simulink model "ACCnovis"  (R2018b)
settings: Solver=ode45  StartTime=0.0  StopTime=80  RelTol=1e-3  EnableMultiTasking=on
values from neighbouring files (symbols this model uses):
  h = 0.9    [initialization.m]
  Kd = 1.2    [initialization.m]
  Kp = 1.5    [initialization.m]
  Lambda1 = 0.5    [initialization.m]
  Lambda2 = 0.7    [initialization.m]
  Lambda3 = 0.75    [initialization.m]
  Lambda4 = 0.7    [initialization.m]
  Lambda5 = 0.7    [initialization.m]
  tau0 = 0.1    [initialization.m]
  tau1 = 0.5    [initialization.m]
  tau2 = 0.7    [initialization.m]
  tau3 = 0.3    [initialization.m]
  tau4 = 0.7    [initialization.m]
  tau5 = 0.9    [initialization.m]
undefined symbols (not defined in the file or in its folder): sigbuilder_block
libraries: simulink x5
settings Model: Creator=apple  LastModifiedBy=ajink
settings DataIOCC: LimitDataPoints=on  SaveFormat=Array
settings OptimizationCC: LifeSpan=inf
settings DebuggingCC: SFUnexpectedBacktrackingDiag=warning  SFNoUnconditionalDefaultTransitionDiag=warning  SFExecutionAtInitializationDiag=none
settings HardwareCC: ProdBitPerPointer=32  ProdBitPerSizeT=32  ProdBitPerPtrDiffT=32  ProdLargestAtomicFloat=None  ProdIntDivRoundTo=Undefined  ProdEndianess=Unspecified  ProdWordSize=32  ProdHWDeviceType=32-bit Generic
settings ModelReferenceCC: PropagateSignalLabelsOutOfModel=off
settings SFSimCC: SimUseLocalCustomCode=off
settings RTWCC: RTWUseLocalCustomCode=off
settings CodeAppCC: StateflowObjectComments=on
settings GRTTargetCC: TargetLangStandard=C89/C90 (ANSI)  GeneratePreprocessorConditionals=Disable all
settings ConfigComp: CovMetricSettings=dw  CovHtmlReporting=on  CovSaveCumulativeToWorkspaceVar=on  CovSaveSingleToWorkspaceVar=on  CovExternalEMLEnable=off

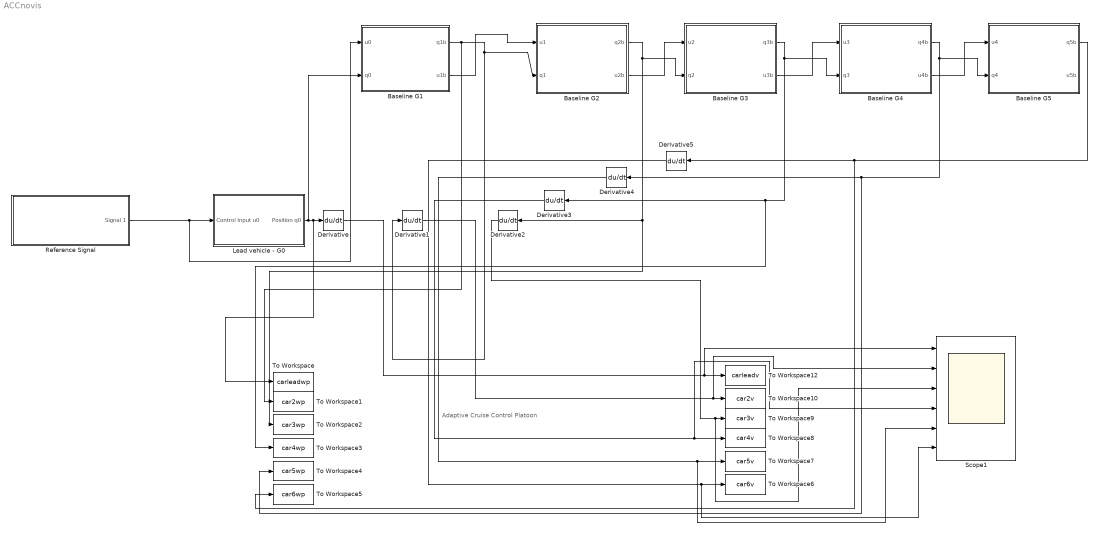
== system ACCnovis ==
  note: Adaptive Cruise Control Platoon
  Baseline G1 : Subsystem
  Baseline G2 : Subsystem
  Baseline G3 : Subsystem
  Baseline G4 : Subsystem
  Baseline G5 : Subsystem
  Derivative{,1..5} (6 alike) : Derivative
  Lead vehicle - G0 : Subsystem
  Reference Signal : Subsystem  Tag=STV Subsys  LoadFcn=sigbuilder_block('load');  StartFcn=sigbuilder_block('start');  StopFcn=sigbuilder_block('stop');  ClipboardFcn=sigbuilder_block('clipboard');  mask(Sigbuilder block){tuvar=[0:10]}
      mask help: Simulink:masks:SigbuilderBlock_MD
      mask init:
      | if ~strcmp(get_param(bdroot(gcbh),'SimulationStatus'),'stopped') tuvar = sigbuilder_block('maskInit'); end
      settings: CopyFcn=sigbuilder_block('copy');  DeleteFcn=sigbuilder_block('delete');  ModelCloseFcn=sigbuilder_block('modelClose');  PreSaveFcn=sigbuilder_block('preSave');  PauseFcn=sigbuilder_block('pause');  ContinueFcn=sigbuilder_block('continue');  NameChangeFcn=sigbuilder_block('namechange');  OpenFcn=sigbuilder_block('open',[6 30 948 639.75 ]);  CloseFcn=sigbuilder_block('close');
      mask Display: plot(0, 0, 100, 100,[2, 2, 32, 32, 2], [68, 8, 8, 68, 68],[32, 2], [38, 38], [32, 19, 2],[53, 60, 44], [32, 17, 17, 2],[16, 16, 31, 31]);txt = getActiveGroup(gcbh);text(2, 100, txt,'verticalAlignment', 'top');
  Scope1 : Scope  NumInputPorts=6
  To Workspace : ToWorkspace  VariableName=carleadwp  SampleTime=-1
      settings: Save2DSignal=2-D array (concatenate along first dimension)
  To Workspace1 : ToWorkspace  VariableName=car2wp  SampleTime=-1
      settings: Save2DSignal=2-D array (concatenate along first dimension)
  To Workspace10 : ToWorkspace  VariableName=car2v  SampleTime=-1
      settings: Save2DSignal=2-D array (concatenate along first dimension)
  To Workspace12 : ToWorkspace  VariableName=carleadv  SampleTime=-1
      settings: Save2DSignal=2-D array (concatenate along first dimension)
  To Workspace2 : ToWorkspace  VariableName=car3wp  SampleTime=-1
      settings: Save2DSignal=2-D array (concatenate along first dimension)
  To Workspace3 : ToWorkspace  VariableName=car4wp  SampleTime=-1
      settings: Save2DSignal=2-D array (concatenate along first dimension)
  To Workspace4 : ToWorkspace  VariableName=car5wp  SampleTime=-1
      settings: Save2DSignal=2-D array (concatenate along first dimension)
  To Workspace5 : ToWorkspace  VariableName=car6wp  SampleTime=-1
      settings: Save2DSignal=2-D array (concatenate along first dimension)
  To Workspace6 : ToWorkspace  VariableName=car6v  SampleTime=-1
      settings: Save2DSignal=2-D array (concatenate along first dimension)
  To Workspace7 : ToWorkspace  VariableName=car5v  SampleTime=-1
      settings: Save2DSignal=2-D array (concatenate along first dimension)
  To Workspace8 : ToWorkspace  VariableName=car4v  SampleTime=-1
      settings: Save2DSignal=2-D array (concatenate along first dimension)
  To Workspace9 : ToWorkspace  VariableName=car3v  SampleTime=-1
      settings: Save2DSignal=2-D array (concatenate along first dimension)
  wires:
  Reference Signal/1(Signal 1) -> Baseline G1/1(u0), Lead vehicle - G0/1(Control Input u0)
  Lead vehicle - G0/1(" Position q0") -> Baseline G1/2(q0), To Workspace/1, Derivative/1
  Baseline G1/1(q1b) -> To Workspace1/1, Baseline G2/2(q1), Derivative1/1
  Derivative/1 -> Scope1/1, To Workspace12/1
  Derivative1/1 -> Scope1/2, To Workspace10/1
  Baseline G1/2(u1b) -> Baseline G2/1(u1)
  Baseline G2/1(q2b) -> To Workspace2/1, Derivative2/1, Baseline G3/2(q2)
  Derivative2/1 -> Scope1/3, To Workspace9/1
  Baseline G2/2(u2b) -> Baseline G3/1(u2)
  Baseline G3/1(q3b) -> Baseline G4/2(q3), To Workspace3/1, Derivative3/1
  Derivative3/1 -> Scope1/4, To Workspace8/1
  Baseline G3/2(u3b) -> Baseline G4/1(u3)
  Baseline G4/1(q4b) -> Baseline G5/2(q4), To Workspace4/1, Derivative4/1
  Derivative4/1 -> Scope1/5, To Workspace7/1
  Baseline G4/2(u4b) -> Baseline G5/1(u4)
  Baseline G5/1(q5b) -> To Workspace5/1, Derivative5/1
  Derivative5/1 -> Scope1/6, To Workspace6/1

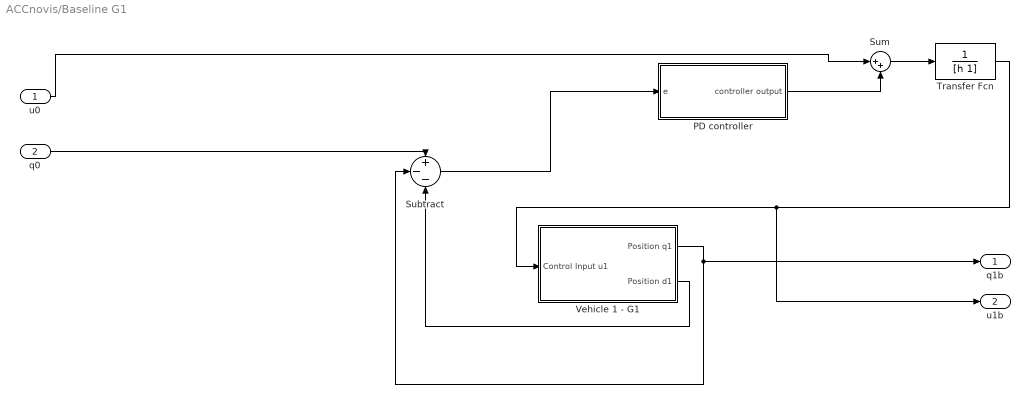
== system ACCnovis/Baseline G1 ==
  u0 : Inport
  q0 : Inport  Port=2
  PD controller : Subsystem
  Subtract : Sum  Inputs=+--
  Sum : Sum  Inputs=|++
  Transfer Fcn : TransferFcn  Denominator=[h 1]
  Vehicle 1 - G1 : Subsystem
  q1b : Outport
  u1b : Outport  Port=2
  wires:
  q0/1 -> Subtract/1
  Subtract/1 -> PD controller/1(e)
  Vehicle 1 - G1/1(" Position q1") -> q1b/1, Subtract/2
  Vehicle 1 - G1/2(" Position d1") -> Subtract/3
  PD controller/1(controller output) -> Sum/2
  Transfer Fcn/1 -> u1b/1, Vehicle 1 - G1/1(Control Input u1)
  Sum/1 -> Transfer Fcn/1
  u0/1 -> Sum/1

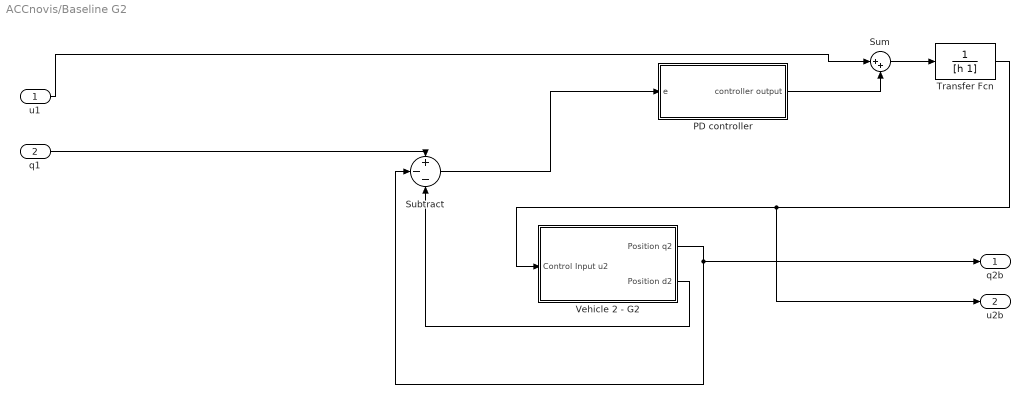
== system ACCnovis/Baseline G2 ==
  u1 : Inport
  q1 : Inport  Port=2
  PD controller : Subsystem
  Subtract : Sum  Inputs=+--
  Sum : Sum  Inputs=|++
  Transfer Fcn : TransferFcn  Denominator=[h 1]
  Vehicle 2 - G2 : Subsystem
  q2b : Outport
  u2b : Outport  Port=2
  wires:
  q1/1 -> Subtract/1
  Subtract/1 -> PD controller/1(e)
  Vehicle 2 - G2/1(" Position q2") -> q2b/1, Subtract/2
  Vehicle 2 - G2/2(" Position d2") -> Subtract/3
  PD controller/1(controller output) -> Sum/2
  Transfer Fcn/1 -> u2b/1, Vehicle 2 - G2/1(Control Input u2)
  Sum/1 -> Transfer Fcn/1
  u1/1 -> Sum/1

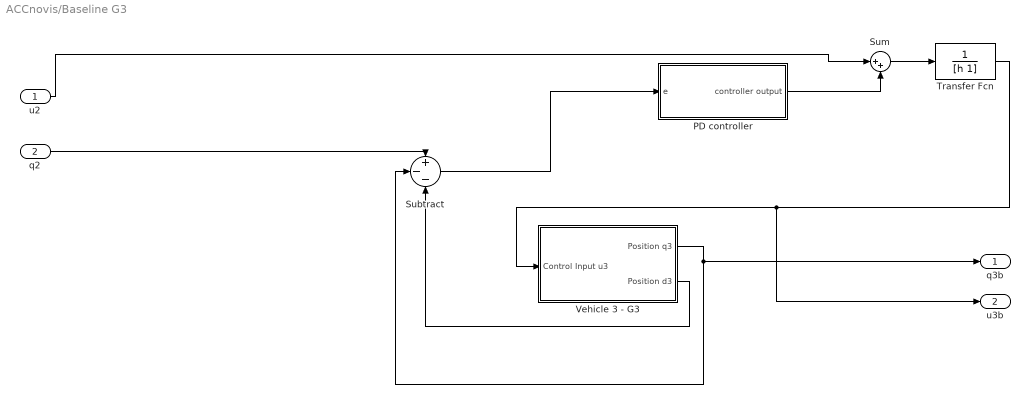
== system ACCnovis/Baseline G3 ==
  u2 : Inport
  q2 : Inport  Port=2
  PD controller : Subsystem
  Subtract : Sum  Inputs=+--
  Sum : Sum  Inputs=|++
  Transfer Fcn : TransferFcn  Denominator=[h 1]
  Vehicle 3 - G3 : Subsystem
  q3b : Outport
  u3b : Outport  Port=2
  wires:
  q2/1 -> Subtract/1
  Subtract/1 -> PD controller/1(e)
  Vehicle 3 - G3/1(" Position q3") -> q3b/1, Subtract/2
  Vehicle 3 - G3/2(" Position d3") -> Subtract/3
  PD controller/1(controller output) -> Sum/2
  Transfer Fcn/1 -> u3b/1, Vehicle 3 - G3/1(Control Input u3)
  Sum/1 -> Transfer Fcn/1
  u2/1 -> Sum/1

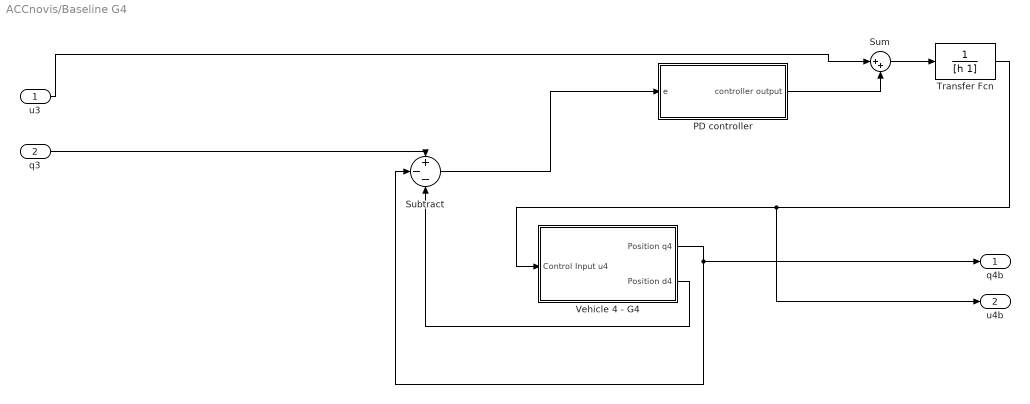
== system ACCnovis/Baseline G4 ==
  u3 : Inport
  q3 : Inport  Port=2
  PD controller : Subsystem
  Subtract : Sum  Inputs=+--
  Sum : Sum  Inputs=|++
  Transfer Fcn : TransferFcn  Denominator=[h 1]
  Vehicle 4 - G4 : Subsystem
  q4b : Outport
  u4b : Outport  Port=2
  wires:
  q3/1 -> Subtract/1
  Subtract/1 -> PD controller/1(e)
  Vehicle 4 - G4/1(" Position q4") -> q4b/1, Subtract/2
  Vehicle 4 - G4/2(" Position d4") -> Subtract/3
  PD controller/1(controller output) -> Sum/2
  Transfer Fcn/1 -> u4b/1, Vehicle 4 - G4/1(Control Input u4)
  Sum/1 -> Transfer Fcn/1
  u3/1 -> Sum/1

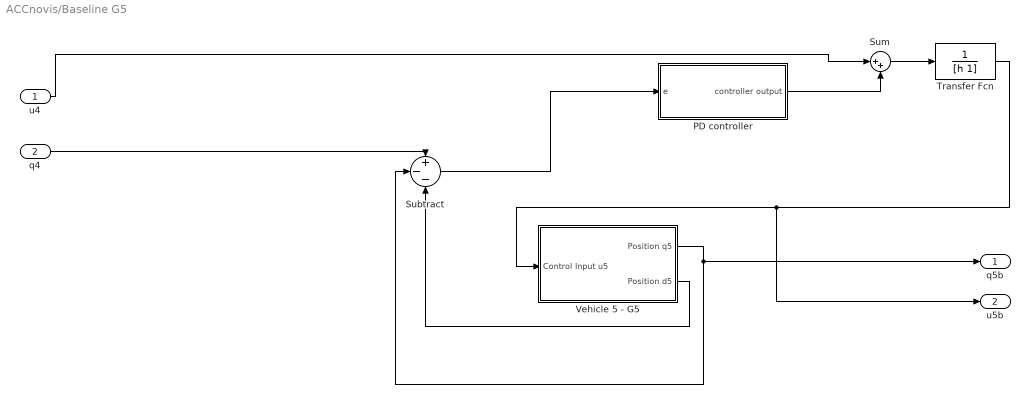
== system ACCnovis/Baseline G5 ==
  u4 : Inport
  q4 : Inport  Port=2
  PD controller : Subsystem
  Subtract : Sum  Inputs=+--
  Sum : Sum  Inputs=|++
  Transfer Fcn : TransferFcn  Denominator=[h 1]
  Vehicle 5 - G5 : Subsystem
  q5b : Outport
  u5b : Outport  Port=2
  wires:
  q4/1 -> Subtract/1
  Subtract/1 -> PD controller/1(e)
  Vehicle 5 - G5/1(" Position q5") -> q5b/1, Subtract/2
  Vehicle 5 - G5/2(" Position d5") -> Subtract/3
  PD controller/1(controller output) -> Sum/2
  Transfer Fcn/1 -> u5b/1, Vehicle 5 - G5/1(Control Input u5)
  Sum/1 -> Transfer Fcn/1
  u4/1 -> Sum/1

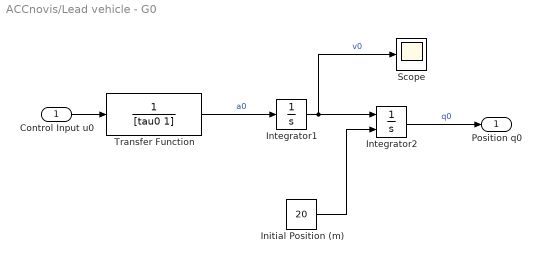
== system ACCnovis/Lead vehicle - G0 ==
  Control Input u0 : Inport
  Initial Position (m) : Constant  Value=20
  Integrator1 : Integrator
  Integrator2 : Integrator  InitialConditionSource=external  InitialCondition=20
  Scope : Scope
  Transfer Function : TransferFcn  Denominator=[tau0 1]
  " Position q0" : Outport
  wires:
  Integrator1/1 -> Scope/1, Integrator2/1  "v0"
  Integrator2/1 -> " Position q0"/1  "q0"
  Initial Position (m)/1 -> Integrator2/2
  Transfer Function/1 -> Integrator1/1  "a0"
  Control Input u0/1 -> Transfer Function/1

== system ACCnovis/Reference Signal ==
  Demux : Demux  Tag=STV Demux  Outputs=1
  FromWs : FromWorkspace  Tag=STV FromWs  VariableName=tuvar  SampleTime=0
      SigBuilderData=|
      | common.afterFinalStr = 'Extrapolate'
      | common.sampleTime = 0
      | dataSet.timeRange = [0 120]
      | dataSet.name = 'Group 1'
      | sbobj.Groups.Name = 'Group 1'
      | sbobj.Groups.Signals.Name = 'Signal 1'
      | sbobj.Groups.Signals.XData = [0 20 20 22.5 22.5 25 50 60 85 110 120]
      | sbobj.Groups.Signals.YData = [0 1.5 -1.5 -1.14 1.75 2 0 0 -2 0 0]
      | sbobj.Groups.TimeRange = [0 120]
  Signal 1 : Outport  Tag=STV Outport
  wires:
  Demux/1 -> Signal 1/1
  FromWs/1 -> Demux/1

== system ACCnovis/Baseline G1/PD controller ==
  e : Inport
  PID Controller : simulink/Continuous/PID Controller  Controller=PID  Form=Parallel  TimeDomain=Continuous-time  SampleTime=-1  IntegratorMethod=Forward Euler  FilterMethod=Forward Euler  ControllerParametersSource=internal  P=Kp  I=0  D=Kd  UseFilter=on  N=100  TunerSelectOption=Transfer Function Based (PID Tuner App)  InitialConditionSource=internal  InitialConditionForIntegrator=0  InitialConditionForFilter=0  DifferentiatorICPrevScaledInput=0  ExternalReset=none  TrackingMode=off  Kt=1  LimitOutput=off  UpperSaturationLimit=inf  LowerSaturationLimit=-inf  LinearizeAsGain=on  AntiWindupMode=none  Kb=1  POutMin=[]  POutMax=[]  IOutMin=[]  IOutMax=[]  DOutMin=[]  DOutMax=[]  NOutMin=[]  NOutMax=[]  SumOutMin=[]  SumOutMax=[]  SaturationOutMin=[]  SaturationOutMax=[]  PParamMin=[]  PParamMax=[]  IParamMin=[]  IParamMax=[]  DParamMin=[]  DParamMax=[]  NParamMin=[]  NParamMax=[]  KbParamMin=[]  KbParamMax=[]  KtParamMin=[]  KtParamMax=[]  KbOutMin=[]  KbOutMax=[]  KtOutMin=[]  KtOutMax=[]  IntegratorOutMin=[]  IntegratorOutMax=[]  FilterOutMin=[]  FilterOutMax=[]  SumI1OutMin=[]  SumI1OutMax=[]  SumI2OutMin=[]  SumI2OutMax=[]  SumI3OutMin=[]  SumI3OutMax=[]  SumI4OutMin=[]  SumI4OutMax=[]  SumDOutMin=[]  SumDOutMax=[]  DifferentiatorOutMin=[]  DifferentiatorOutMax=[]  FilterDiffOutCoefMin=[]  FilterDiffOutCoefMax=[]  ReciprocalOutMin=[]  ReciprocalOutMax=[]  SumDenOutMin=[]  SumDenOutMax=[]  SumNumOutMin=[]  SumNumOutMax=[]  DivideOutMin=[]  DivideOutMax=[]  IntegratorContinuousStateAttributes=''  IntegratorStateMustResolveToSignalObject=off  IntegratorRTWStateStorageClass=Auto  FilterContinuousStateAttributes=''  FilterStateMustResolveToSignalObject=off  FilterRTWStateStorageClass=Auto  ParallelPVariant=InternalParameters  IdealPVariant=Disabled  IVariant=InternalParameters  DVariant=InternalParameters  IntegratorVariant=Continuous  SatVariant=Disabled  AWVariant=Passthrough  PCopyVariant=Disabled  TRVariant=Disabled  FdbkBlocksVariant=Forward  IdealPFdbkVariant=Disabled  SatFdbkVariant=Disabled  DerivativeFilterVariant=ContFilter  NVariant=InternalParameters  NCopyVariant=Disabled  FilterICVariant=InternalICsFilter  IntegratorICVariant=InternalICs  ExternalResetVariant=Disabled  TRSumVariant=Passthrough  SumFdbkVariant=Disabled  SumVariant=Sum_PID
  controller output : Outport
  wires:
  PID Controller/1 -> controller output/1
  e/1 -> PID Controller/1

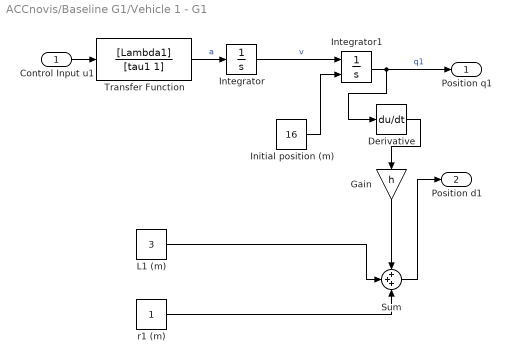
== system ACCnovis/Baseline G1/Vehicle 1 - G1 ==
  Control Input u1 : Inport
  Derivative : Derivative
  Gain : Gain  Gain=h
  Initial position (m) : Constant  Value=16
  Integrator : Integrator
  Integrator1 : Integrator  InitialConditionSource=external  InitialCondition=20
  L1 (m) : Constant  Value=3
  Sum : Sum  Inputs=3
  Transfer Function : TransferFcn  Numerator=[Lambda1]  Denominator=[tau1 1]
  r1 (m) : Constant
  " Position q1" : Outport
  " Position d1" : Outport  Port=2
  wires:
  Integrator1/1 -> Derivative/1, " Position q1"/1  "q1"
  Initial position (m)/1 -> Integrator1/2
  Transfer Function/1 -> Integrator/1  "a"
  Integrator/1 -> Integrator1/1  "v"
  Control Input u1/1 -> Transfer Function/1
  L1 (m)/1 -> Sum/2
  r1 (m)/1 -> Sum/3
  Sum/1 -> " Position d1"/1
  Derivative/1 -> Gain/1
  Gain/1 -> Sum/1

== system ACCnovis/Baseline G2/PD controller ==
  e : Inport
  PID Controller : simulink/Continuous/PID Controller  Controller=PID  Form=Parallel  TimeDomain=Continuous-time  SampleTime=-1  IntegratorMethod=Forward Euler  FilterMethod=Forward Euler  ControllerParametersSource=internal  P=Kp  I=0  D=Kd  UseFilter=on  N=100  TunerSelectOption=Transfer Function Based (PID Tuner App)  InitialConditionSource=internal  InitialConditionForIntegrator=0  InitialConditionForFilter=0  DifferentiatorICPrevScaledInput=0  ExternalReset=none  TrackingMode=off  Kt=1  LimitOutput=off  UpperSaturationLimit=inf  LowerSaturationLimit=-inf  LinearizeAsGain=on  AntiWindupMode=none  Kb=1  POutMin=[]  POutMax=[]  IOutMin=[]  IOutMax=[]  DOutMin=[]  DOutMax=[]  NOutMin=[]  NOutMax=[]  SumOutMin=[]  SumOutMax=[]  SaturationOutMin=[]  SaturationOutMax=[]  PParamMin=[]  PParamMax=[]  IParamMin=[]  IParamMax=[]  DParamMin=[]  DParamMax=[]  NParamMin=[]  NParamMax=[]  KbParamMin=[]  KbParamMax=[]  KtParamMin=[]  KtParamMax=[]  KbOutMin=[]  KbOutMax=[]  KtOutMin=[]  KtOutMax=[]  IntegratorOutMin=[]  IntegratorOutMax=[]  FilterOutMin=[]  FilterOutMax=[]  SumI1OutMin=[]  SumI1OutMax=[]  SumI2OutMin=[]  SumI2OutMax=[]  SumI3OutMin=[]  SumI3OutMax=[]  SumI4OutMin=[]  SumI4OutMax=[]  SumDOutMin=[]  SumDOutMax=[]  DifferentiatorOutMin=[]  DifferentiatorOutMax=[]  FilterDiffOutCoefMin=[]  FilterDiffOutCoefMax=[]  ReciprocalOutMin=[]  ReciprocalOutMax=[]  SumDenOutMin=[]  SumDenOutMax=[]  SumNumOutMin=[]  SumNumOutMax=[]  DivideOutMin=[]  DivideOutMax=[]  IntegratorContinuousStateAttributes=''  IntegratorStateMustResolveToSignalObject=off  IntegratorRTWStateStorageClass=Auto  FilterContinuousStateAttributes=''  FilterStateMustResolveToSignalObject=off  FilterRTWStateStorageClass=Auto  ParallelPVariant=InternalParameters  IdealPVariant=Disabled  IVariant=InternalParameters  DVariant=InternalParameters  IntegratorVariant=Continuous  SatVariant=Disabled  AWVariant=Passthrough  PCopyVariant=Disabled  TRVariant=Disabled  FdbkBlocksVariant=Forward  IdealPFdbkVariant=Disabled  SatFdbkVariant=Disabled  DerivativeFilterVariant=ContFilter  NVariant=InternalParameters  NCopyVariant=Disabled  FilterICVariant=InternalICsFilter  IntegratorICVariant=InternalICs  ExternalResetVariant=Disabled  TRSumVariant=Passthrough  SumFdbkVariant=Disabled  SumVariant=Sum_PID
  controller output : Outport
  wires:
  PID Controller/1 -> controller output/1
  e/1 -> PID Controller/1

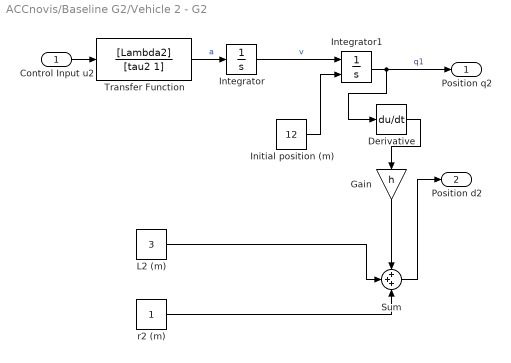
== system ACCnovis/Baseline G2/Vehicle 2 - G2 ==
  Control Input u2 : Inport
  Derivative : Derivative
  Gain : Gain  Gain=h
  Initial position (m) : Constant  Value=12
  Integrator : Integrator
  Integrator1 : Integrator  InitialConditionSource=external  InitialCondition=20
  L2 (m) : Constant  Value=3
  Sum : Sum  Inputs=3
  Transfer Function : TransferFcn  Numerator=[Lambda2]  Denominator=[tau2 1]
  r2 (m) : Constant
  " Position q2" : Outport
  " Position d2" : Outport  Port=2
  wires:
  Integrator1/1 -> Derivative/1, " Position q2"/1  "q1"
  Initial position (m)/1 -> Integrator1/2
  Transfer Function/1 -> Integrator/1  "a"
  Integrator/1 -> Integrator1/1  "v"
  Control Input u2/1 -> Transfer Function/1
  L2 (m)/1 -> Sum/2
  r2 (m)/1 -> Sum/3
  Sum/1 -> " Position d2"/1
  Derivative/1 -> Gain/1
  Gain/1 -> Sum/1

== system ACCnovis/Baseline G3/PD controller ==
  e : Inport
  PID Controller : simulink/Continuous/PID Controller  Controller=PID  Form=Parallel  TimeDomain=Continuous-time  SampleTime=-1  IntegratorMethod=Forward Euler  FilterMethod=Forward Euler  ControllerParametersSource=internal  P=Kp  I=0  D=Kd  UseFilter=on  N=100  TunerSelectOption=Transfer Function Based (PID Tuner App)  InitialConditionSource=internal  InitialConditionForIntegrator=0  InitialConditionForFilter=0  DifferentiatorICPrevScaledInput=0  ExternalReset=none  TrackingMode=off  Kt=1  LimitOutput=off  UpperSaturationLimit=inf  LowerSaturationLimit=-inf  LinearizeAsGain=on  AntiWindupMode=none  Kb=1  POutMin=[]  POutMax=[]  IOutMin=[]  IOutMax=[]  DOutMin=[]  DOutMax=[]  NOutMin=[]  NOutMax=[]  SumOutMin=[]  SumOutMax=[]  SaturationOutMin=[]  SaturationOutMax=[]  PParamMin=[]  PParamMax=[]  IParamMin=[]  IParamMax=[]  DParamMin=[]  DParamMax=[]  NParamMin=[]  NParamMax=[]  KbParamMin=[]  KbParamMax=[]  KtParamMin=[]  KtParamMax=[]  KbOutMin=[]  KbOutMax=[]  KtOutMin=[]  KtOutMax=[]  IntegratorOutMin=[]  IntegratorOutMax=[]  FilterOutMin=[]  FilterOutMax=[]  SumI1OutMin=[]  SumI1OutMax=[]  SumI2OutMin=[]  SumI2OutMax=[]  SumI3OutMin=[]  SumI3OutMax=[]  SumI4OutMin=[]  SumI4OutMax=[]  SumDOutMin=[]  SumDOutMax=[]  DifferentiatorOutMin=[]  DifferentiatorOutMax=[]  FilterDiffOutCoefMin=[]  FilterDiffOutCoefMax=[]  ReciprocalOutMin=[]  ReciprocalOutMax=[]  SumDenOutMin=[]  SumDenOutMax=[]  SumNumOutMin=[]  SumNumOutMax=[]  DivideOutMin=[]  DivideOutMax=[]  IntegratorContinuousStateAttributes=''  IntegratorStateMustResolveToSignalObject=off  IntegratorRTWStateStorageClass=Auto  FilterContinuousStateAttributes=''  FilterStateMustResolveToSignalObject=off  FilterRTWStateStorageClass=Auto  ParallelPVariant=InternalParameters  IdealPVariant=Disabled  IVariant=InternalParameters  DVariant=InternalParameters  IntegratorVariant=Continuous  SatVariant=Disabled  AWVariant=Passthrough  PCopyVariant=Disabled  TRVariant=Disabled  FdbkBlocksVariant=Forward  IdealPFdbkVariant=Disabled  SatFdbkVariant=Disabled  DerivativeFilterVariant=ContFilter  NVariant=InternalParameters  NCopyVariant=Disabled  FilterICVariant=InternalICsFilter  IntegratorICVariant=InternalICs  ExternalResetVariant=Disabled  TRSumVariant=Passthrough  SumFdbkVariant=Disabled  SumVariant=Sum_PID
  controller output : Outport
  wires:
  PID Controller/1 -> controller output/1
  e/1 -> PID Controller/1

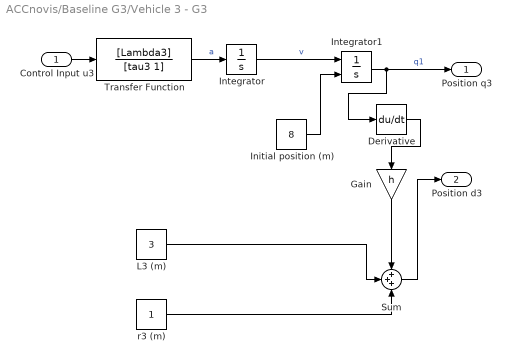
== system ACCnovis/Baseline G3/Vehicle 3 - G3 ==
  Control Input u3 : Inport
  Derivative : Derivative
  Gain : Gain  Gain=h
  Initial position (m) : Constant  Value=8
  Integrator : Integrator
  Integrator1 : Integrator  InitialConditionSource=external  InitialCondition=20
  L3 (m) : Constant  Value=3
  Sum : Sum  Inputs=3
  Transfer Function : TransferFcn  Numerator=[Lambda3]  Denominator=[tau3 1]
  r3 (m) : Constant
  " Position q3" : Outport
  " Position d3" : Outport  Port=2
  wires:
  Integrator1/1 -> Derivative/1, " Position q3"/1  "q1"
  Initial position (m)/1 -> Integrator1/2
  Transfer Function/1 -> Integrator/1  "a"
  Integrator/1 -> Integrator1/1  "v"
  Control Input u3/1 -> Transfer Function/1
  L3 (m)/1 -> Sum/2
  r3 (m)/1 -> Sum/3
  Sum/1 -> " Position d3"/1
  Derivative/1 -> Gain/1
  Gain/1 -> Sum/1

== system ACCnovis/Baseline G4/PD controller ==
  e : Inport
  PID Controller : simulink/Continuous/PID Controller  Controller=PID  Form=Parallel  TimeDomain=Continuous-time  SampleTime=-1  IntegratorMethod=Forward Euler  FilterMethod=Forward Euler  ControllerParametersSource=internal  P=Kp  I=0  D=Kd  UseFilter=on  N=100  TunerSelectOption=Transfer Function Based (PID Tuner App)  InitialConditionSource=internal  InitialConditionForIntegrator=0  InitialConditionForFilter=0  DifferentiatorICPrevScaledInput=0  ExternalReset=none  TrackingMode=off  Kt=1  LimitOutput=off  UpperSaturationLimit=inf  LowerSaturationLimit=-inf  LinearizeAsGain=on  AntiWindupMode=none  Kb=1  POutMin=[]  POutMax=[]  IOutMin=[]  IOutMax=[]  DOutMin=[]  DOutMax=[]  NOutMin=[]  NOutMax=[]  SumOutMin=[]  SumOutMax=[]  SaturationOutMin=[]  SaturationOutMax=[]  PParamMin=[]  PParamMax=[]  IParamMin=[]  IParamMax=[]  DParamMin=[]  DParamMax=[]  NParamMin=[]  NParamMax=[]  KbParamMin=[]  KbParamMax=[]  KtParamMin=[]  KtParamMax=[]  KbOutMin=[]  KbOutMax=[]  KtOutMin=[]  KtOutMax=[]  IntegratorOutMin=[]  IntegratorOutMax=[]  FilterOutMin=[]  FilterOutMax=[]  SumI1OutMin=[]  SumI1OutMax=[]  SumI2OutMin=[]  SumI2OutMax=[]  SumI3OutMin=[]  SumI3OutMax=[]  SumI4OutMin=[]  SumI4OutMax=[]  SumDOutMin=[]  SumDOutMax=[]  DifferentiatorOutMin=[]  DifferentiatorOutMax=[]  FilterDiffOutCoefMin=[]  FilterDiffOutCoefMax=[]  ReciprocalOutMin=[]  ReciprocalOutMax=[]  SumDenOutMin=[]  SumDenOutMax=[]  SumNumOutMin=[]  SumNumOutMax=[]  DivideOutMin=[]  DivideOutMax=[]  IntegratorContinuousStateAttributes=''  IntegratorStateMustResolveToSignalObject=off  IntegratorRTWStateStorageClass=Auto  FilterContinuousStateAttributes=''  FilterStateMustResolveToSignalObject=off  FilterRTWStateStorageClass=Auto  ParallelPVariant=InternalParameters  IdealPVariant=Disabled  IVariant=InternalParameters  DVariant=InternalParameters  IntegratorVariant=Continuous  SatVariant=Disabled  AWVariant=Passthrough  PCopyVariant=Disabled  TRVariant=Disabled  FdbkBlocksVariant=Forward  IdealPFdbkVariant=Disabled  SatFdbkVariant=Disabled  DerivativeFilterVariant=ContFilter  NVariant=InternalParameters  NCopyVariant=Disabled  FilterICVariant=InternalICsFilter  IntegratorICVariant=InternalICs  ExternalResetVariant=Disabled  TRSumVariant=Passthrough  SumFdbkVariant=Disabled  SumVariant=Sum_PID
  controller output : Outport
  wires:
  PID Controller/1 -> controller output/1
  e/1 -> PID Controller/1

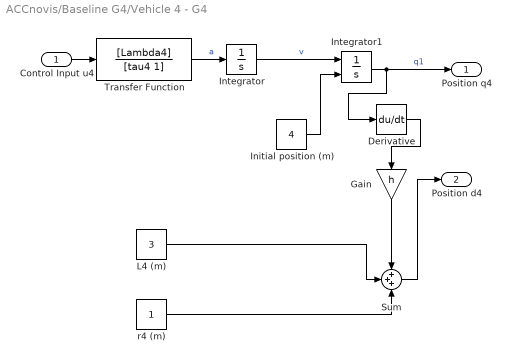
== system ACCnovis/Baseline G4/Vehicle 4 - G4 ==
  Control Input u4 : Inport
  Derivative : Derivative
  Gain : Gain  Gain=h
  Initial position (m) : Constant  Value=4
  Integrator : Integrator
  Integrator1 : Integrator  InitialConditionSource=external  InitialCondition=20
  L4 (m) : Constant  Value=3
  Sum : Sum  Inputs=3
  Transfer Function : TransferFcn  Numerator=[Lambda4]  Denominator=[tau4 1]
  r4 (m) : Constant
  " Position q4" : Outport
  " Position d4" : Outport  Port=2
  wires:
  Integrator1/1 -> Derivative/1, " Position q4"/1  "q1"
  Initial position (m)/1 -> Integrator1/2
  Transfer Function/1 -> Integrator/1  "a"
  Integrator/1 -> Integrator1/1  "v"
  Control Input u4/1 -> Transfer Function/1
  L4 (m)/1 -> Sum/2
  r4 (m)/1 -> Sum/3
  Sum/1 -> " Position d4"/1
  Derivative/1 -> Gain/1
  Gain/1 -> Sum/1

== system ACCnovis/Baseline G5/PD controller ==
  e : Inport
  PID Controller : simulink/Continuous/PID Controller  Controller=PID  Form=Parallel  TimeDomain=Continuous-time  SampleTime=-1  IntegratorMethod=Forward Euler  FilterMethod=Forward Euler  ControllerParametersSource=internal  P=Kp  I=0  D=Kd  UseFilter=on  N=100  TunerSelectOption=Transfer Function Based (PID Tuner App)  InitialConditionSource=internal  InitialConditionForIntegrator=0  InitialConditionForFilter=0  DifferentiatorICPrevScaledInput=0  ExternalReset=none  TrackingMode=off  Kt=1  LimitOutput=off  UpperSaturationLimit=inf  LowerSaturationLimit=-inf  LinearizeAsGain=on  AntiWindupMode=none  Kb=1  POutMin=[]  POutMax=[]  IOutMin=[]  IOutMax=[]  DOutMin=[]  DOutMax=[]  NOutMin=[]  NOutMax=[]  SumOutMin=[]  SumOutMax=[]  SaturationOutMin=[]  SaturationOutMax=[]  PParamMin=[]  PParamMax=[]  IParamMin=[]  IParamMax=[]  DParamMin=[]  DParamMax=[]  NParamMin=[]  NParamMax=[]  KbParamMin=[]  KbParamMax=[]  KtParamMin=[]  KtParamMax=[]  KbOutMin=[]  KbOutMax=[]  KtOutMin=[]  KtOutMax=[]  IntegratorOutMin=[]  IntegratorOutMax=[]  FilterOutMin=[]  FilterOutMax=[]  SumI1OutMin=[]  SumI1OutMax=[]  SumI2OutMin=[]  SumI2OutMax=[]  SumI3OutMin=[]  SumI3OutMax=[]  SumI4OutMin=[]  SumI4OutMax=[]  SumDOutMin=[]  SumDOutMax=[]  DifferentiatorOutMin=[]  DifferentiatorOutMax=[]  FilterDiffOutCoefMin=[]  FilterDiffOutCoefMax=[]  ReciprocalOutMin=[]  ReciprocalOutMax=[]  SumDenOutMin=[]  SumDenOutMax=[]  SumNumOutMin=[]  SumNumOutMax=[]  DivideOutMin=[]  DivideOutMax=[]  IntegratorContinuousStateAttributes=''  IntegratorStateMustResolveToSignalObject=off  IntegratorRTWStateStorageClass=Auto  FilterContinuousStateAttributes=''  FilterStateMustResolveToSignalObject=off  FilterRTWStateStorageClass=Auto  ParallelPVariant=InternalParameters  IdealPVariant=Disabled  IVariant=InternalParameters  DVariant=InternalParameters  IntegratorVariant=Continuous  SatVariant=Disabled  AWVariant=Passthrough  PCopyVariant=Disabled  TRVariant=Disabled  FdbkBlocksVariant=Forward  IdealPFdbkVariant=Disabled  SatFdbkVariant=Disabled  DerivativeFilterVariant=ContFilter  NVariant=InternalParameters  NCopyVariant=Disabled  FilterICVariant=InternalICsFilter  IntegratorICVariant=InternalICs  ExternalResetVariant=Disabled  TRSumVariant=Passthrough  SumFdbkVariant=Disabled  SumVariant=Sum_PID
  controller output : Outport
  wires:
  PID Controller/1 -> controller output/1
  e/1 -> PID Controller/1

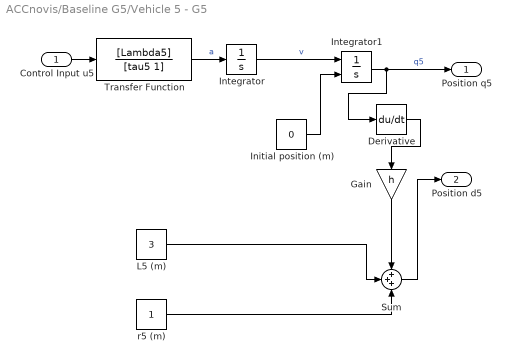
== system ACCnovis/Baseline G5/Vehicle 5 - G5 ==
  Control Input u5 : Inport
  Derivative : Derivative
  Gain : Gain  Gain=h
  Initial position (m) : Constant  Value=0
  Integrator : Integrator
  Integrator1 : Integrator  InitialConditionSource=external  InitialCondition=20
  L5 (m) : Constant  Value=3
  Sum : Sum  Inputs=3
  Transfer Function : TransferFcn  Numerator=[Lambda5]  Denominator=[tau5 1]
  r5 (m) : Constant
  " Position q5" : Outport
  " Position d5" : Outport  Port=2
  wires:
  Integrator1/1 -> Derivative/1, " Position q5"/1  "q5"
  Initial position (m)/1 -> Integrator1/2
  Transfer Function/1 -> Integrator/1  "a"
  Integrator/1 -> Integrator1/1  "v"
  Control Input u5/1 -> Transfer Function/1
  L5 (m)/1 -> Sum/2
  r5 (m)/1 -> Sum/3
  Sum/1 -> " Position d5"/1
  Derivative/1 -> Gain/1
  Gain/1 -> Sum/1
